simulink subsystem "Point3S"  (R2023a)
settings: Solver=VariableStepAuto  StartTime=0.0  StopTime=10.0  RelTol=1e-3
undefined symbols (not defined in the file): magnitude
settings Model: Creator=bjmyn  LastModifiedBy=bjmyn

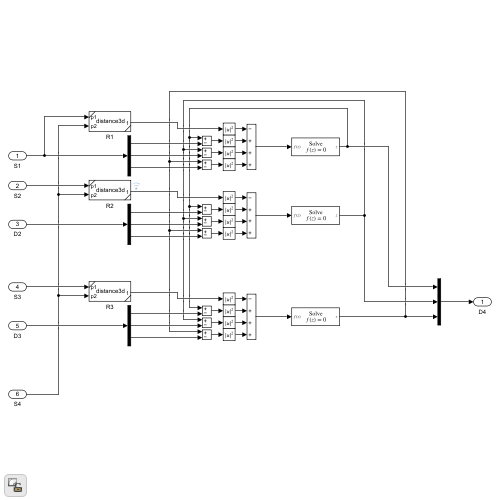
[thumbnail: Simulink's stored preview of the top-level diagram]
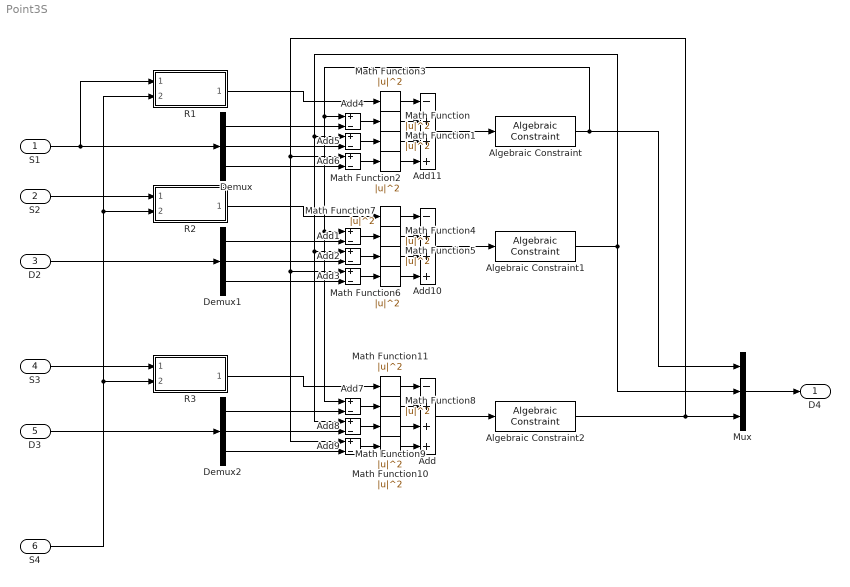
== system Point3S ==
  S1 : Inport
  S2 : Inport  Port=2
  D2 : Inport  Port=3
  S3 : Inport  Port=4
  D3 : Inport  Port=5
  S4 : Inport  Port=6
  Add : Sum  Inputs=-+++
  Add{1..9} (9 alike) : Sum  Inputs=+-
  Add10 : Sum  Inputs=-+++
  Add11 : Sum  Inputs=-+++
  Algebraic Constraint : AlgebraicConstraint
  Algebraic Constraint1 : AlgebraicConstraint  InitialGuess=460
  Algebraic Constraint2 : AlgebraicConstraint  InitialGuess=380
  Demux : Demux  Outputs=3
  Demux1 : Demux  Outputs=3
  Demux2 : Demux  Outputs=3
  Math Function{,1..11} (12 alike) : Math  Operator=magnitude^2
  Mux : Mux  Inputs=3
  R1 : Subsystem  ReferencedSubsystem=distance3d
  R2 : Subsystem  ReferencedSubsystem=distance3d
  R3 : Subsystem  ReferencedSubsystem=distance3d
  D4 : Outport
  wires:
  S1/1 -> Demux/1, R1/1
  S2/1 -> R2/1
  D3/1 -> Demux2/1
  S4/1 -> R3/2, R2/2, R1/2
  S3/1 -> R3/1
  Demux1/1 -> Add1/2
  Demux1/2 -> Add2/2
  Demux1/3 -> Add3/2
  Demux/3 -> Add6/2
  Demux/2 -> Add5/2
  Demux/1 -> Add4/2
  Demux2/3 -> Add9/2
  Demux2/2 -> Add8/2
  Demux2/1 -> Add7/2
  Add4/1 -> Math Function/1
  Math Function/1 -> Add11/2
  Math Function1/1 -> Add11/3
  Add5/1 -> Math Function1/1
  Math Function2/1 -> Add11/4
  Add6/1 -> Math Function2/1
  Math Function3/1 -> Add11/1
  R1/1 -> Math Function3/1
  R2/1 -> Math Function7/1
  Math Function7/1 -> Add10/1
  Add3/1 -> Math Function6/1
  Math Function6/1 -> Add10/4
  Add2/1 -> Math Function5/1
  Math Function5/1 -> Add10/3
  Math Function4/1 -> Add10/2
  Add1/1 -> Math Function4/1
  Add7/1 -> Math Function8/1
  Math Function8/1 -> Add/2
  Math Function9/1 -> Add/3
  Add8/1 -> Math Function9/1
  Math Function10/1 -> Add/4
  Add9/1 -> Math Function10/1
  Math Function11/1 -> Add/1
  R3/1 -> Math Function11/1
  Add11/1 -> Algebraic Constraint/1
  Add10/1 -> Algebraic Constraint1/1
  Add/1 -> Algebraic Constraint2/1
  Mux/1 -> D4/1
  Algebraic Constraint/1 -> Mux/1, Add4/1, Add1/1, Add7/1
  Algebraic Constraint1/1 -> Mux/2, Add5/1, Add2/1, Add8/1
  Algebraic Constraint2/1 -> Mux/3, Add6/1, Add3/1, Add9/1
  D2/1 -> Demux1/1
